simulink model "wamjc7"  (Simulink 8.3)
settings: Solver=ode4  SolverMode=SingleTasking  StartTime=0.0  StopTime=inf  FixedStep=sample_time  RelTol=1e-3
undefined symbols (not defined in the file): arm_home, arm_home_norest, arm_j2mt, arm_m2jp, b, bit, C, CAN_init, enc_per_rev, FT_init, hand_on, MT_init, puck_I_per_Nm, rotFT2Hand, sample_time, Standard, VL1_init, VL2_init
libraries: xpclib x43, simulink x27, xpcutilitieslib x6, dspmathops x1, dspadpt3 x1, dspindex x1, dspbuff3 x1
(part 5 of 5)

== matlab function Subsystem/Impedance Controller/Subsystem1/Dynamics Compensation1 ==
  data: hand_on input double; tau output double; q input double; qd input double; qdd input double; FTsensor output double
function [tau, FTsensor] = dynamicsComp(hand_on,q,qd,qdd)
%-------------------------------------------------------------------------------------
%   SETUP THE ARM
%-------------------------------------------------------------------------------------    
    DH_a = [0 0 0.045 -0.045 0 0 0];
    DH_d = [0 0 .55 0 0.3 0 0.061];
    DH_alpha = [-pi/2 pi/2 -pi/2 pi/2 -pi/2 pi/2 0];

    m = [8.3936 4.8487 1.7251 2.17266212 0.35655692 0.40915886 0.07548270];
    
    com = zeros(3,7);
    com(:,1) = [0.3506e-3, 132.6795e-3, 0.6286e-3];
    com(:,2) = [-0.2230e-3, -21.3924e-3, 13.3754e-3];
    com(:,3) = [-38.7565e-3, 217.9078e-3, 0.0252e-3];
    com(:,4) = [0.00553408,0.00006822,0.11927695];
    com(:,5) = [0.00005483,0.02886286,0.00148493];
    com(:,6) = [-0.00005923,-0.01686123,0.02419052];
    com(:,7) = [ 0.00014836,0.00007252,-0.00335185];
    
    % Need Inertia matricies
    I = zeros(3,3,7);
    I(:,:,1) = [ 95157.4294e-6,   246.1404e-6,   -95.0183e-6 ;
                   246.1404e-6, 92032.3524e-6,  -962.6725e-6 ;
                   -95.0183e-6,  -962.6725e-6, 59290.5997e-6 ];
    I(:,:,2) = [ 29326.8098e-6,   -43.3994e-6,  -129.2942e-6 ;
                   -43.3994e-6, 20781.5826e-6,  1348.6924e-6 ;
                  -129.2942e-6,  1348.6924e-6, 22807.3271e-6 ];
    I(:,:,3) = [ 56662.2970e-6, -2321.6892e-6,     8.2125e-6 ;
                 -2321.6892e-6,  3158.0509e-6,   -16.6307e-6 ;
                     8.2125e-6,   -16.6307e-6, 56806.6024e-6 ];
    I(:,:,4) = [  0.01067491,  0.00004503, -0.00135557 ;
                  0.00004503,  0.01058659, -0.00011002 ;
                 -0.00135557, -0.00011002,  0.00282036 ];
    I(:,:,5) = [  0.00037112, -0.00000008, -0.00000003 ;
                 -0.00000008,  0.00019434, -0.00001613 ;
                 -0.00000003, -0.00001613,  0.00038209 ];
    I(:,:,6) =  [  0.00054889,  0.00000019, -0.00000010 ;
                   0.00000019,  0.00023846, -0.00004430 ;
                  -0.00000010, -0.00004430,  0.00045133 ];
    I(:,:,7) = [ 0.00003911, 0.00000019, 0.00000000 ;      % WAM without hand
                 0.00000019, 0.00003877, 0.00000000 ;
                 0.00000000, 0.00000000, 0.00007614 ];
    
    %Link Gear Ratio
    % The differential drive mechanism was ignored here because it's not
    % supported by the robotic toolbox yet.
    % Please refer to: http://www.me.unm.edu/~starr/research/WAM_MassParams_AA-00.pdf
    G = zeros(7,1);
    G(1) =  42.00;
    G(2) =  28.25;
    G(3) =  28.25;
    G(4) =  18.00;
    G(5) =  9.70;
    G(6) =  9.70;
    G(7) =  14.93;
    %Link Motor Inertia
    Jm = zeros(7,1);
    Jm(1) = 0.00011631;
    Jm(2) = 0.00011831;
    Jm(3) = 0.00011831;
    Jm(4) = 0.00010686;
    Jm(5) = 0.00001685;
    Jm(6) = 0.00001745;
    Jm(7) = 0.00000142;
             
    if hand_on
        hand_mass = 1.3731;
        DH_d(7) = DH_d(7) + .0953; % Adding the distance to the hand frame for the Schunk Gripper
        com(:,7) = ([0.001127;	-0.000211;	0.054851].*hand_mass + com(:,7).*m(7))/(hand_mass + m(7)); % Finding the combined center of mass
        m(7) = m(7) + hand_mass; % Adding the mass of the hand
        I(:,:,7) = [ .003167342,          0,         0;       % Approximate Inertia Tensor for Schunk Gripper
                              0, .001128942,         0;
                              0,          0, .00258007;];
    end
    
%-------------------------------------------------------------------------------------
%  END SETUP OF THE ARM
%-------------------------------------------------------------------------------------

    z0 = [0;0;1];
    grav = [0 0 9.81];
	fext = zeros(6, 1);
    n = 7;
    FTsensor = zeros(6,1);
    
    tau = zeros(n,1);
    
    Fm = zeros(3,7);
    Nm = zeros(3,7);
    N = zeros(3,1);
    pstarm = zeros(3,7);
    Rm = zeros(3,3,7);
    w = zeros(3,1);
    wd = zeros(3,1);
    v = zeros(3,1);
    vd = grav(:);
    
    
    %
	% init some variables, compute the link rotation matrices
	%
    for j=1:n,
        a = DH_a(j);
        d = DH_d(j);
        alpha = DH_alpha(j);
        Tj = getTransformDH(a, d, alpha, q(j));
        
        pstar = [a; d*sin(alpha); d*cos(alpha)];
        if j == 1,
            pstar = eye(3) * pstar;
            Tj = eye(4) * Tj;
        end
        pstarm(:,j) = pstar;
        Rm(:,:,j) = Tj(1:3,1:3);
    end
    
    %
	%  the forward recursion
	%
    for j=1:n,
        Rt = Rm(:,:,j)';	% transpose!!
        pstar = pstarm(:,j);
        r = com(:,j)';

        %
        % statement order is important here
        %
        % revolute axis
        wd = Rt*(wd + z0*qdd(j) + cross(w,z0*qd(j)));
        w = Rt*(w + z0*qd(j));
        %v = cross(w,pstar) + Rt*v;
        vd = cross(wd,pstar) + cross(w, cross(w,pstar)) + Rt*vd;

        %vhat = cross(wd,r') + cross(w,cross(w,r')) + vd;
        vhat = cross(wd,r') + cross(w,cross(w,r')) + vd;
        F = m(j)*vhat;
        N = I(1:3,1:3,j)*wd + cross(w,I(1:3,1:3,j)*w);
        Fm(:,j) = F;
        Nm(:,j) = N;
    end
    
    
    %
	%  the backward recursion
	%

    fext = fext(:);
    f = fext(1:3);		% force/moments on end of arm
    nn = fext(4:6);

    for j=n:-1:1,
        pstar = pstarm(:,j);

        %
        % order of these statements is important, since both
        % nn and f are functions of previous f.
        %
        if j == n,
            R = eye(3,3);
        else
            R = Rm(:,:,j+1);
        end
        r = com(:,j)';
        
        % The expected force/torque at the sensor.  Used for dynamic compensation
        % of the gripper.
        if j == n
            FTsensor(1:3) = R*f + Fm(:,j);
            FTsensor(4:6) = cross(r',Fm(:,j));
        end
        
        nn = R*(nn + cross(R'*pstar,f)) + cross(pstar+r',Fm(:,j)) + Nm(:,j);
        f = R*f + Fm(:,j);
        
        R = Rm(:,:,j);
        % revolute
        tau(j) = nn'*(R'*z0) + G(j)^2 * Jm(j)*qdd(j);% + abs(G(j)) * friction(link, qd(j));
    end

end

function T = getTransformDH(a,d,alpha,q)
    ct = cos(q);
    st = sin(q);
    cb = cos(alpha);
    sb = sin(alpha);
    
    T = [ ct, -st*cb,  st*sb, a*ct;
          st,  ct*cb, -ct*sb, a*st;
          0, sb, cb, d;
          0, 0, 0, 1 ];
end

== matlab function Subsystem/Impedance Controller/Subsystem1/Dynamics Compensation2 ==
  data: hand_on input double; tau output double; q input double; qd input double; qdd input double; FTsensor output double
function [tau, FTsensor] = dynamicsComp(hand_on,q,qd,qdd)
%-------------------------------------------------------------------------------------
%   SETUP THE ARM
%-------------------------------------------------------------------------------------    
    DH_a = [0 0 0.045 -0.045 0 0 0];
    DH_d = [0 0 .55 0 0.3 0 0.061];
    DH_alpha = [-pi/2 pi/2 -pi/2 pi/2 -pi/2 pi/2 0];

    m = [8.3936 4.8487 1.7251 2.17266212 0.35655692 0.40915886 0.07548270];
    
    com = zeros(3,7);
    com(:,1) = [0.3506e-3, 132.6795e-3, 0.6286e-3];
    com(:,2) = [-0.2230e-3, -21.3924e-3, 13.3754e-3];
    com(:,3) = [-38.7565e-3, 217.9078e-3, 0.0252e-3];
    com(:,4) = [0.00553408,0.00006822,0.11927695];
    com(:,5) = [0.00005483,0.02886286,0.00148493];
    com(:,6) = [-0.00005923,-0.01686123,0.02419052];
    com(:,7) = [ 0.00014836,0.00007252,-0.00335185];
    
    % Need Inertia matricies
    I = zeros(3,3,7);
    I(:,:,1) = [ 95157.4294e-6,   246.1404e-6,   -95.0183e-6 ;
                   246.1404e-6, 92032.3524e-6,  -962.6725e-6 ;
                   -95.0183e-6,  -962.6725e-6, 59290.5997e-6 ];
    I(:,:,2) = [ 29326.8098e-6,   -43.3994e-6,  -129.2942e-6 ;
                   -43.3994e-6, 20781.5826e-6,  1348.6924e-6 ;
                  -129.2942e-6,  1348.6924e-6, 22807.3271e-6 ];
    I(:,:,3) = [ 56662.2970e-6, -2321.6892e-6,     8.2125e-6 ;
                 -2321.6892e-6,  3158.0509e-6,   -16.6307e-6 ;
                     8.2125e-6,   -16.6307e-6, 56806.6024e-6 ];
    I(:,:,4) = [  0.01067491,  0.00004503, -0.00135557 ;
                  0.00004503,  0.01058659, -0.00011002 ;
                 -0.00135557, -0.00011002,  0.00282036 ];
    I(:,:,5) = [  0.00037112, -0.00000008, -0.00000003 ;
                 -0.00000008,  0.00019434, -0.00001613 ;
                 -0.00000003, -0.00001613,  0.00038209 ];
    I(:,:,6) =  [  0.00054889,  0.00000019, -0.00000010 ;
                   0.00000019,  0.00023846, -0.00004430 ;
                  -0.00000010, -0.00004430,  0.00045133 ];
    I(:,:,7) = [ 0.00003911, 0.00000019, 0.00000000 ;      % WAM without hand
                 0.00000019, 0.00003877, 0.00000000 ;
                 0.00000000, 0.00000000, 0.00007614 ];
    
    %Link Gear Ratio
    % The differential drive mechanism was ignored here because it's not
    % supported by the robotic toolbox yet.
    % Please refer to: http://www.me.unm.edu/~starr/research/WAM_MassParams_AA-00.pdf
    G = zeros(7,1);
    G(1) =  42.00;
    G(2) =  28.25;
    G(3) =  28.25;
    G(4) =  18.00;
    G(5) =  9.70;
    G(6) =  9.70;
    G(7) =  14.93;
    %Link Motor Inertia
    Jm = zeros(7,1);
    Jm(1) = 0.00011631;
    Jm(2) = 0.00011831;
    Jm(3) = 0.00011831;
    Jm(4) = 0.00010686;
    Jm(5) = 0.00001685;
    Jm(6) = 0.00001745;
    Jm(7) = 0.00000142;
             
    if hand_on
        hand_mass = 1.3731;
        DH_d(7) = DH_d(7) + .0953; % Adding the distance to the hand frame for the Schunk Gripper
        com(:,7) = ([0.001127;	-0.000211;	0.054851].*hand_mass + com(:,7).*m(7))/(hand_mass + m(7)); % Finding the combined center of mass
        m(7) = m(7) + hand_mass; % Adding the mass of the hand
        I(:,:,7) = [ .003167342,          0,         0;       % Approximate Inertia Tensor for Schunk Gripper
                              0, .001128942,         0;
                              0,          0, .00258007;];
    end
    
%-------------------------------------------------------------------------------------
%  END SETUP OF THE ARM
%-------------------------------------------------------------------------------------

    z0 = [0;0;1];
    grav = [0 0 9.81];
	fext = zeros(6, 1);
    n = 7;
    FTsensor = zeros(6,1);
    
    tau = zeros(n,1);
    
    Fm = zeros(3,7);
    Nm = zeros(3,7);
    N = zeros(3,1);
    pstarm = zeros(3,7);
    Rm = zeros(3,3,7);
    w = zeros(3,1);
    wd = zeros(3,1);
    v = zeros(3,1);
    vd = grav(:);
    
    
    %
	% init some variables, compute the link rotation matrices
	%
    for j=1:n,
        a = DH_a(j);
        d = DH_d(j);
        alpha = DH_alpha(j);
        Tj = getTransformDH(a, d, alpha, q(j));
        
        pstar = [a; d*sin(alpha); d*cos(alpha)];
        if j == 1,
            pstar = eye(3) * pstar;
            Tj = eye(4) * Tj;
        end
        pstarm(:,j) = pstar;
        Rm(:,:,j) = Tj(1:3,1:3);
    end
    
    %
	%  the forward recursion
	%
    for j=1:n,
        Rt = Rm(:,:,j)';	% transpose!!
        pstar = pstarm(:,j);
        r = com(:,j)';

        %
        % statement order is important here
        %
        % revolute axis
        wd = Rt*(wd + z0*qdd(j) + cross(w,z0*qd(j)));
        w = Rt*(w + z0*qd(j));
        %v = cross(w,pstar) + Rt*v;
        vd = cross(wd,pstar) + cross(w, cross(w,pstar)) + Rt*vd;

        %vhat = cross(wd,r') + cross(w,cross(w,r')) + vd;
        vhat = cross(wd,r') + cross(w,cross(w,r')) + vd;
        F = m(j)*vhat;
        N = I(1:3,1:3,j)*wd + cross(w,I(1:3,1:3,j)*w);
        Fm(:,j) = F;
        Nm(:,j) = N;
    end
    
    
    %
	%  the backward recursion
	%

    fext = fext(:);
    f = fext(1:3);		% force/moments on end of arm
    nn = fext(4:6);

    for j=n:-1:1,
        pstar = pstarm(:,j);

        %
        % order of these statements is important, since both
        % nn and f are functions of previous f.
        %
        if j == n,
            R = eye(3,3);
        else
            R = Rm(:,:,j+1);
        end
        r = com(:,j)';
        
        % The expected force/torque at the sensor.  Used for dynamic compensation
        % of the gripper.
        if j == n
            FTsensor(1:3) = R*f + Fm(:,j);
            FTsensor(4:6) = cross(r',Fm(:,j));
        end
        
        nn = R*(nn + cross(R'*pstar,f)) + cross(pstar+r',Fm(:,j)) + Nm(:,j);
        f = R*f + Fm(:,j);
        
        R = Rm(:,:,j);
        % revolute
        tau(j) = nn'*(R'*z0) + G(j)^2 * Jm(j)*qdd(j);% + abs(G(j)) * friction(link, qd(j));
    end

end

function T = getTransformDH(a,d,alpha,q)
    ct = cos(q);
    st = sin(q);
    cb = cos(alpha);
    sb = sin(alpha);
    
    T = [ ct, -st*cb,  st*sb, a*ct;
          st,  ct*cb, -ct*sb, a*st;
          0, sb, cb, d;
          0, 0, 0, 1 ];
end

== matlab function Subsystem/Impedance Controller/Subsystem1/Dynamics Compensation3 ==
  data: hand_on input double; tau output double; q input double; qd input double; qdd input double; FTsensor output double
function [tau, FTsensor] = dynamicsComp(hand_on,q,qd,qdd)
%-------------------------------------------------------------------------------------
%   SETUP THE ARM
%-------------------------------------------------------------------------------------    
    DH_a = [0 0 0.045 -0.045 0 0 0];
    DH_d = [0 0 .55 0 0.3 0 0.061];
    DH_alpha = [-pi/2 pi/2 -pi/2 pi/2 -pi/2 pi/2 0];

    m = [8.3936 4.8487 1.7251 2.17266212 0.35655692 0.40915886 0.07548270];
    
    com = zeros(3,7);
    com(:,1) = [0.3506e-3, 132.6795e-3, 0.6286e-3];
    com(:,2) = [-0.2230e-3, -21.3924e-3, 13.3754e-3];
    com(:,3) = [-38.7565e-3, 217.9078e-3, 0.0252e-3];
    com(:,4) = [0.00553408,0.00006822,0.11927695];
    com(:,5) = [0.00005483,0.02886286,0.00148493];
    com(:,6) = [-0.00005923,-0.01686123,0.02419052];
    com(:,7) = [ 0.00014836,0.00007252,-0.00335185];
    
    % Need Inertia matricies
    I = zeros(3,3,7);
    I(:,:,1) = [ 95157.4294e-6,   246.1404e-6,   -95.0183e-6 ;
                   246.1404e-6, 92032.3524e-6,  -962.6725e-6 ;
                   -95.0183e-6,  -962.6725e-6, 59290.5997e-6 ];
    I(:,:,2) = [ 29326.8098e-6,   -43.3994e-6,  -129.2942e-6 ;
                   -43.3994e-6, 20781.5826e-6,  1348.6924e-6 ;
                  -129.2942e-6,  1348.6924e-6, 22807.3271e-6 ];
    I(:,:,3) = [ 56662.2970e-6, -2321.6892e-6,     8.2125e-6 ;
                 -2321.6892e-6,  3158.0509e-6,   -16.6307e-6 ;
                     8.2125e-6,   -16.6307e-6, 56806.6024e-6 ];
    I(:,:,4) = [  0.01067491,  0.00004503, -0.00135557 ;
                  0.00004503,  0.01058659, -0.00011002 ;
                 -0.00135557, -0.00011002,  0.00282036 ];
    I(:,:,5) = [  0.00037112, -0.00000008, -0.00000003 ;
                 -0.00000008,  0.00019434, -0.00001613 ;
                 -0.00000003, -0.00001613,  0.00038209 ];
    I(:,:,6) =  [  0.00054889,  0.00000019, -0.00000010 ;
                   0.00000019,  0.00023846, -0.00004430 ;
                  -0.00000010, -0.00004430,  0.00045133 ];
    I(:,:,7) = [ 0.00003911, 0.00000019, 0.00000000 ;      % WAM without hand
                 0.00000019, 0.00003877, 0.00000000 ;
                 0.00000000, 0.00000000, 0.00007614 ];
    
    %Link Gear Ratio
    % The differential drive mechanism was ignored here because it's not
    % supported by the robotic toolbox yet.
    % Please refer to: http://www.me.unm.edu/~starr/research/WAM_MassParams_AA-00.pdf
    G = zeros(7,1);
    G(1) =  42.00;
    G(2) =  28.25;
    G(3) =  28.25;
    G(4) =  18.00;
    G(5) =  9.70;
    G(6) =  9.70;
    G(7) =  14.93;
    %Link Motor Inertia
    Jm = zeros(7,1);
    Jm(1) = 0.00011631;
    Jm(2) = 0.00011831;
    Jm(3) = 0.00011831;
    Jm(4) = 0.00010686;
    Jm(5) = 0.00001685;
    Jm(6) = 0.00001745;
    Jm(7) = 0.00000142;
             
    if hand_on
        hand_mass = 1.3731;
        DH_d(7) = DH_d(7) + .0953; % Adding the distance to the hand frame for the Schunk Gripper
        com(:,7) = ([0.001127;	-0.000211;	0.054851].*hand_mass + com(:,7).*m(7))/(hand_mass + m(7)); % Finding the combined center of mass
        m(7) = m(7) + hand_mass; % Adding the mass of the hand
        I(:,:,7) = [ .003167342,          0,         0;       % Approximate Inertia Tensor for Schunk Gripper
                              0, .001128942,         0;
                              0,          0, .00258007;];
    end
    
%-------------------------------------------------------------------------------------
%  END SETUP OF THE ARM
%-------------------------------------------------------------------------------------

    z0 = [0;0;1];
    grav = [0 0 9.81];
	fext = zeros(6, 1);
    n = 7;
    FTsensor = zeros(6,1);
    
    tau = zeros(n,1);
    
    Fm = zeros(3,7);
    Nm = zeros(3,7);
    N = zeros(3,1);
    pstarm = zeros(3,7);
    Rm = zeros(3,3,7);
    w = zeros(3,1);
    wd = zeros(3,1);
    v = zeros(3,1);
    vd = grav(:);
    
    
    %
	% init some variables, compute the link rotation matrices
	%
    for j=1:n,
        a = DH_a(j);
        d = DH_d(j);
        alpha = DH_alpha(j);
        Tj = getTransformDH(a, d, alpha, q(j));
        
        pstar = [a; d*sin(alpha); d*cos(alpha)];
        if j == 1,
            pstar = eye(3) * pstar;
            Tj = eye(4) * Tj;
        end
        pstarm(:,j) = pstar;
        Rm(:,:,j) = Tj(1:3,1:3);
    end
    
    %
	%  the forward recursion
	%
    for j=1:n,
        Rt = Rm(:,:,j)';	% transpose!!
        pstar = pstarm(:,j);
        r = com(:,j)';

        %
        % statement order is important here
        %
        % revolute axis
        wd = Rt*(wd + z0*qdd(j) + cross(w,z0*qd(j)));
        w = Rt*(w + z0*qd(j));
        %v = cross(w,pstar) + Rt*v;
        vd = cross(wd,pstar) + cross(w, cross(w,pstar)) + Rt*vd;

        %vhat = cross(wd,r') + cross(w,cross(w,r')) + vd;
        vhat = cross(wd,r') + cross(w,cross(w,r')) + vd;
        F = m(j)*vhat;
        N = I(1:3,1:3,j)*wd + cross(w,I(1:3,1:3,j)*w);
        Fm(:,j) = F;
        Nm(:,j) = N;
    end
    
    
    %
	%  the backward recursion
	%

    fext = fext(:);
    f = fext(1:3);		% force/moments on end of arm
    nn = fext(4:6);

    for j=n:-1:1,
        pstar = pstarm(:,j);

        %
        % order of these statements is important, since both
        % nn and f are functions of previous f.
        %
        if j == n,
            R = eye(3,3);
        else
            R = Rm(:,:,j+1);
        end
        r = com(:,j)';
        
        % The expected force/torque at the sensor.  Used for dynamic compensation
        % of the gripper.
        if j == n
            FTsensor(1:3) = R*f + Fm(:,j);
            FTsensor(4:6) = cross(r',Fm(:,j));
        end
        
        nn = R*(nn + cross(R'*pstar,f)) + cross(pstar+r',Fm(:,j)) + Nm(:,j);
        f = R*f + Fm(:,j);
        
        R = Rm(:,:,j);
        % revolute
        tau(j) = nn'*(R'*z0) + G(j)^2 * Jm(j)*qdd(j);% + abs(G(j)) * friction(link, qd(j));
    end

end

function T = getTransformDH(a,d,alpha,q)
    ct = cos(q);
    st = sin(q);
    cb = cos(alpha);
    sb = sin(alpha);
    
    T = [ ct, -st*cb,  st*sb, a*ct;
          st,  ct*cb, -ct*sb, a*st;
          0, sb, cb, d;
          0, 0, 0, 1 ];
end

== matlab function Subsystem/Impedance Controller/Subsystem1/Dynamics Compensation4 ==
  data: hand_on input double; tau output double; q input double; qd input double; qdd input double; FTsensor output double
function [tau, FTsensor] = dynamicsComp(hand_on,q,qd,qdd)
%-------------------------------------------------------------------------------------
%   SETUP THE ARM
%-------------------------------------------------------------------------------------    
    DH_a = [0 0 0.045 -0.045 0 0 0];
    DH_d = [0 0 .55 0 0.3 0 0.061];
    DH_alpha = [-pi/2 pi/2 -pi/2 pi/2 -pi/2 pi/2 0];

    m = [8.3936 4.8487 1.7251 2.17266212 0.35655692 0.40915886 0.07548270];
    
    com = zeros(3,7);
    com(:,1) = [0.3506e-3, 132.6795e-3, 0.6286e-3];
    com(:,2) = [-0.2230e-3, -21.3924e-3, 13.3754e-3];
    com(:,3) = [-38.7565e-3, 217.9078e-3, 0.0252e-3];
    com(:,4) = [0.00553408,0.00006822,0.11927695];
    com(:,5) = [0.00005483,0.02886286,0.00148493];
    com(:,6) = [-0.00005923,-0.01686123,0.02419052];
    com(:,7) = [ 0.00014836,0.00007252,-0.00335185];
    
    % Need Inertia matricies
    I = zeros(3,3,7);
    I(:,:,1) = [ 95157.4294e-6,   246.1404e-6,   -95.0183e-6 ;
                   246.1404e-6, 92032.3524e-6,  -962.6725e-6 ;
                   -95.0183e-6,  -962.6725e-6, 59290.5997e-6 ];
    I(:,:,2) = [ 29326.8098e-6,   -43.3994e-6,  -129.2942e-6 ;
                   -43.3994e-6, 20781.5826e-6,  1348.6924e-6 ;
                  -129.2942e-6,  1348.6924e-6, 22807.3271e-6 ];
    I(:,:,3) = [ 56662.2970e-6, -2321.6892e-6,     8.2125e-6 ;
                 -2321.6892e-6,  3158.0509e-6,   -16.6307e-6 ;
                     8.2125e-6,   -16.6307e-6, 56806.6024e-6 ];
    I(:,:,4) = [  0.01067491,  0.00004503, -0.00135557 ;
                  0.00004503,  0.01058659, -0.00011002 ;
                 -0.00135557, -0.00011002,  0.00282036 ];
    I(:,:,5) = [  0.00037112, -0.00000008, -0.00000003 ;
                 -0.00000008,  0.00019434, -0.00001613 ;
                 -0.00000003, -0.00001613,  0.00038209 ];
    I(:,:,6) =  [  0.00054889,  0.00000019, -0.00000010 ;
                   0.00000019,  0.00023846, -0.00004430 ;
                  -0.00000010, -0.00004430,  0.00045133 ];
    I(:,:,7) = [ 0.00003911, 0.00000019, 0.00000000 ;      % WAM without hand
                 0.00000019, 0.00003877, 0.00000000 ;
                 0.00000000, 0.00000000, 0.00007614 ];
    
    %Link Gear Ratio
    % The differential drive mechanism was ignored here because it's not
    % supported by the robotic toolbox yet.
    % Please refer to: http://www.me.unm.edu/~starr/research/WAM_MassParams_AA-00.pdf
    G = zeros(7,1);
    G(1) =  42.00;
    G(2) =  28.25;
    G(3) =  28.25;
    G(4) =  18.00;
    G(5) =  9.70;
    G(6) =  9.70;
    G(7) =  14.93;
    %Link Motor Inertia
    Jm = zeros(7,1);
    Jm(1) = 0.00011631;
    Jm(2) = 0.00011831;
    Jm(3) = 0.00011831;
    Jm(4) = 0.00010686;
    Jm(5) = 0.00001685;
    Jm(6) = 0.00001745;
    Jm(7) = 0.00000142;
             
    if hand_on
        hand_mass = 1.3731;
        DH_d(7) = DH_d(7) + .0953; % Adding the distance to the hand frame for the Schunk Gripper
        com(:,7) = ([0.001127;	-0.000211;	0.054851].*hand_mass + com(:,7).*m(7))/(hand_mass + m(7)); % Finding the combined center of mass
        m(7) = m(7) + hand_mass; % Adding the mass of the hand
        I(:,:,7) = [ .003167342,          0,         0;       % Approximate Inertia Tensor for Schunk Gripper
                              0, .001128942,         0;
                              0,          0, .00258007;];
    end
    
%-------------------------------------------------------------------------------------
%  END SETUP OF THE ARM
%-------------------------------------------------------------------------------------

    z0 = [0;0;1];
    grav = [0 0 9.81];
	fext = zeros(6, 1);
    n = 7;
    FTsensor = zeros(6,1);
    
    tau = zeros(n,1);
    
    Fm = zeros(3,7);
    Nm = zeros(3,7);
    N = zeros(3,1);
    pstarm = zeros(3,7);
    Rm = zeros(3,3,7);
    w = zeros(3,1);
    wd = zeros(3,1);
    v = zeros(3,1);
    vd = grav(:);
    
    
    %
	% init some variables, compute the link rotation matrices
	%
    for j=1:n,
        a = DH_a(j);
        d = DH_d(j);
        alpha = DH_alpha(j);
        Tj = getTransformDH(a, d, alpha, q(j));
        
        pstar = [a; d*sin(alpha); d*cos(alpha)];
        if j == 1,
            pstar = eye(3) * pstar;
            Tj = eye(4) * Tj;
        end
        pstarm(:,j) = pstar;
        Rm(:,:,j) = Tj(1:3,1:3);
    end
    
    %
	%  the forward recursion
	%
    for j=1:n,
        Rt = Rm(:,:,j)';	% transpose!!
        pstar = pstarm(:,j);
        r = com(:,j)';

        %
        % statement order is important here
        %
        % revolute axis
        wd = Rt*(wd + z0*qdd(j) + cross(w,z0*qd(j)));
        w = Rt*(w + z0*qd(j));
        %v = cross(w,pstar) + Rt*v;
        vd = cross(wd,pstar) + cross(w, cross(w,pstar)) + Rt*vd;

        %vhat = cross(wd,r') + cross(w,cross(w,r')) + vd;
        vhat = cross(wd,r') + cross(w,cross(w,r')) + vd;
        F = m(j)*vhat;
        N = I(1:3,1:3,j)*wd + cross(w,I(1:3,1:3,j)*w);
        Fm(:,j) = F;
        Nm(:,j) = N;
    end
    
    
    %
	%  the backward recursion
	%

    fext = fext(:);
    f = fext(1:3);		% force/moments on end of arm
    nn = fext(4:6);

    for j=n:-1:1,
        pstar = pstarm(:,j);

        %
        % order of these statements is important, since both
        % nn and f are functions of previous f.
        %
        if j == n,
            R = eye(3,3);
        else
            R = Rm(:,:,j+1);
        end
        r = com(:,j)';
        
        % The expected force/torque at the sensor.  Used for dynamic compensation
        % of the gripper.
        if j == n
            FTsensor(1:3) = R*f + Fm(:,j);
            FTsensor(4:6) = cross(r',Fm(:,j));
        end
        
        nn = R*(nn + cross(R'*pstar,f)) + cross(pstar+r',Fm(:,j)) + Nm(:,j);
        f = R*f + Fm(:,j);
        
        R = Rm(:,:,j);
        % revolute
        tau(j) = nn'*(R'*z0) + G(j)^2 * Jm(j)*qdd(j);% + abs(G(j)) * friction(link, qd(j));
    end

end

function T = getTransformDH(a,d,alpha,q)
    ct = cos(q);
    st = sin(q);
    cb = cos(alpha);
    sb = sin(alpha);
    
    T = [ ct, -st*cb,  st*sb, a*ct;
          st,  ct*cb, -ct*sb, a*st;
          0, sb, cb, d;
          0, 0, 0, 1 ];
end

== matlab function Subsystem/Impedance Controller/Subsystem1/Dynamics Compensation5 ==
  data: hand_on input double; tau output double; q input double; qd input double; qdd input double; FTsensor output double
function [tau, FTsensor] = dynamicsComp(hand_on,q,qd,qdd)
%-------------------------------------------------------------------------------------
%   SETUP THE ARM
%-------------------------------------------------------------------------------------    
    DH_a = [0 0 0.045 -0.045 0 0 0];
    DH_d = [0 0 .55 0 0.3 0 0.061];
    DH_alpha = [-pi/2 pi/2 -pi/2 pi/2 -pi/2 pi/2 0];

    m = [8.3936 4.8487 1.7251 2.17266212 0.35655692 0.40915886 0.07548270];
    
    com = zeros(3,7);
    com(:,1) = [0.3506e-3, 132.6795e-3, 0.6286e-3];
    com(:,2) = [-0.2230e-3, -21.3924e-3, 13.3754e-3];
    com(:,3) = [-38.7565e-3, 217.9078e-3, 0.0252e-3];
    com(:,4) = [0.00553408,0.00006822,0.11927695];
    com(:,5) = [0.00005483,0.02886286,0.00148493];
    com(:,6) = [-0.00005923,-0.01686123,0.02419052];
    com(:,7) = [ 0.00014836,0.00007252,-0.00335185];
    
    % Need Inertia matricies
    I = zeros(3,3,7);
    I(:,:,1) = [ 95157.4294e-6,   246.1404e-6,   -95.0183e-6 ;
                   246.1404e-6, 92032.3524e-6,  -962.6725e-6 ;
                   -95.0183e-6,  -962.6725e-6, 59290.5997e-6 ];
    I(:,:,2) = [ 29326.8098e-6,   -43.3994e-6,  -129.2942e-6 ;
                   -43.3994e-6, 20781.5826e-6,  1348.6924e-6 ;
                  -129.2942e-6,  1348.6924e-6, 22807.3271e-6 ];
    I(:,:,3) = [ 56662.2970e-6, -2321.6892e-6,     8.2125e-6 ;
                 -2321.6892e-6,  3158.0509e-6,   -16.6307e-6 ;
                     8.2125e-6,   -16.6307e-6, 56806.6024e-6 ];
    I(:,:,4) = [  0.01067491,  0.00004503, -0.00135557 ;
                  0.00004503,  0.01058659, -0.00011002 ;
                 -0.00135557, -0.00011002,  0.00282036 ];
    I(:,:,5) = [  0.00037112, -0.00000008, -0.00000003 ;
                 -0.00000008,  0.00019434, -0.00001613 ;
                 -0.00000003, -0.00001613,  0.00038209 ];
    I(:,:,6) =  [  0.00054889,  0.00000019, -0.00000010 ;
                   0.00000019,  0.00023846, -0.00004430 ;
                  -0.00000010, -0.00004430,  0.00045133 ];
    I(:,:,7) = [ 0.00003911, 0.00000019, 0.00000000 ;      % WAM without hand
                 0.00000019, 0.00003877, 0.00000000 ;
                 0.00000000, 0.00000000, 0.00007614 ];
    
    %Link Gear Ratio
    % The differential drive mechanism was ignored here because it's not
    % supported by the robotic toolbox yet.
    % Please refer to: http://www.me.unm.edu/~starr/research/WAM_MassParams_AA-00.pdf
    G = zeros(7,1);
    G(1) =  42.00;
    G(2) =  28.25;
    G(3) =  28.25;
    G(4) =  18.00;
    G(5) =  9.70;
    G(6) =  9.70;
    G(7) =  14.93;
    %Link Motor Inertia
    Jm = zeros(7,1);
    Jm(1) = 0.00011631;
    Jm(2) = 0.00011831;
    Jm(3) = 0.00011831;
    Jm(4) = 0.00010686;
    Jm(5) = 0.00001685;
    Jm(6) = 0.00001745;
    Jm(7) = 0.00000142;
             
    if hand_on
        hand_mass = 1.3731;
        DH_d(7) = DH_d(7) + .0953; % Adding the distance to the hand frame for the Schunk Gripper
        com(:,7) = ([0.001127;	-0.000211;	0.054851].*hand_mass + com(:,7).*m(7))/(hand_mass + m(7)); % Finding the combined center of mass
        m(7) = m(7) + hand_mass; % Adding the mass of the hand
        I(:,:,7) = [ .003167342,          0,         0;       % Approximate Inertia Tensor for Schunk Gripper
                              0, .001128942,         0;
                              0,          0, .00258007;];
    end
    
%-------------------------------------------------------------------------------------
%  END SETUP OF THE ARM
%-------------------------------------------------------------------------------------

    z0 = [0;0;1];
    grav = [0 0 9.81];
	fext = zeros(6, 1);
    n = 7;
    FTsensor = zeros(6,1);
    
    tau = zeros(n,1);
    
    Fm = zeros(3,7);
    Nm = zeros(3,7);
    N = zeros(3,1);
    pstarm = zeros(3,7);
    Rm = zeros(3,3,7);
    w = zeros(3,1);
    wd = zeros(3,1);
    v = zeros(3,1);
    vd = grav(:);
    
    
    %
	% init some variables, compute the link rotation matrices
	%
    for j=1:n,
        a = DH_a(j);
        d = DH_d(j);
        alpha = DH_alpha(j);
        Tj = getTransformDH(a, d, alpha, q(j));
        
        pstar = [a; d*sin(alpha); d*cos(alpha)];
        if j == 1,
            pstar = eye(3) * pstar;
            Tj = eye(4) * Tj;
        end
        pstarm(:,j) = pstar;
        Rm(:,:,j) = Tj(1:3,1:3);
    end
    
    %
	%  the forward recursion
	%
    for j=1:n,
        Rt = Rm(:,:,j)';	% transpose!!
        pstar = pstarm(:,j);
        r = com(:,j)';

        %
        % statement order is important here
        %
        % revolute axis
        wd = Rt*(wd + z0*qdd(j) + cross(w,z0*qd(j)));
        w = Rt*(w + z0*qd(j));
        %v = cross(w,pstar) + Rt*v;
        vd = cross(wd,pstar) + cross(w, cross(w,pstar)) + Rt*vd;

        %vhat = cross(wd,r') + cross(w,cross(w,r')) + vd;
        vhat = cross(wd,r') + cross(w,cross(w,r')) + vd;
        F = m(j)*vhat;
        N = I(1:3,1:3,j)*wd + cross(w,I(1:3,1:3,j)*w);
        Fm(:,j) = F;
        Nm(:,j) = N;
    end
    
    
    %
	%  the backward recursion
	%

    fext = fext(:);
    f = fext(1:3);		% force/moments on end of arm
    nn = fext(4:6);

    for j=n:-1:1,
        pstar = pstarm(:,j);

        %
        % order of these statements is important, since both
        % nn and f are functions of previous f.
        %
        if j == n,
            R = eye(3,3);
        else
            R = Rm(:,:,j+1);
        end
        r = com(:,j)';
        
        % The expected force/torque at the sensor.  Used for dynamic compensation
        % of the gripper.
        if j == n
            FTsensor(1:3) = R*f + Fm(:,j);
            FTsensor(4:6) = cross(r',Fm(:,j));
        end
        
        nn = R*(nn + cross(R'*pstar,f)) + cross(pstar+r',Fm(:,j)) + Nm(:,j);
        f = R*f + Fm(:,j);
        
        R = Rm(:,:,j);
        % revolute
        tau(j) = nn'*(R'*z0) + G(j)^2 * Jm(j)*qdd(j);% + abs(G(j)) * friction(link, qd(j));
    end

end

function T = getTransformDH(a,d,alpha,q)
    ct = cos(q);
    st = sin(q);
    cb = cos(alpha);
    sb = sin(alpha);
    
    T = [ ct, -st*cb,  st*sb, a*ct;
          st,  ct*cb, -ct*sb, a*st;
          0, sb, cb, d;
          0, 0, 0, 1 ];
end

== matlab function Subsystem/Impedance Controller/Subsystem1/Dynamics Compensation6 ==
  data: hand_on input double; tau output double; q input double; qd input double; qdd input double; FTsensor output double
function [tau, FTsensor] = dynamicsComp(hand_on,q,qd,qdd)
%-------------------------------------------------------------------------------------
%   SETUP THE ARM
%-------------------------------------------------------------------------------------    
    DH_a = [0 0 0.045 -0.045 0 0 0];
    DH_d = [0 0 .55 0 0.3 0 0.061];
    DH_alpha = [-pi/2 pi/2 -pi/2 pi/2 -pi/2 pi/2 0];

    m = [8.3936 4.8487 1.7251 2.17266212 0.35655692 0.40915886 0.07548270];
    
    com = zeros(3,7);
    com(:,1) = [0.3506e-3, 132.6795e-3, 0.6286e-3];
    com(:,2) = [-0.2230e-3, -21.3924e-3, 13.3754e-3];
    com(:,3) = [-38.7565e-3, 217.9078e-3, 0.0252e-3];
    com(:,4) = [0.00553408,0.00006822,0.11927695];
    com(:,5) = [0.00005483,0.02886286,0.00148493];
    com(:,6) = [-0.00005923,-0.01686123,0.02419052];
    com(:,7) = [ 0.00014836,0.00007252,-0.00335185];
    
    % Need Inertia matricies
    I = zeros(3,3,7);
    I(:,:,1) = [ 95157.4294e-6,   246.1404e-6,   -95.0183e-6 ;
                   246.1404e-6, 92032.3524e-6,  -962.6725e-6 ;
                   -95.0183e-6,  -962.6725e-6, 59290.5997e-6 ];
    I(:,:,2) = [ 29326.8098e-6,   -43.3994e-6,  -129.2942e-6 ;
                   -43.3994e-6, 20781.5826e-6,  1348.6924e-6 ;
                  -129.2942e-6,  1348.6924e-6, 22807.3271e-6 ];
    I(:,:,3) = [ 56662.2970e-6, -2321.6892e-6,     8.2125e-6 ;
                 -2321.6892e-6,  3158.0509e-6,   -16.6307e-6 ;
                     8.2125e-6,   -16.6307e-6, 56806.6024e-6 ];
    I(:,:,4) = [  0.01067491,  0.00004503, -0.00135557 ;
                  0.00004503,  0.01058659, -0.00011002 ;
                 -0.00135557, -0.00011002,  0.00282036 ];
    I(:,:,5) = [  0.00037112, -0.00000008, -0.00000003 ;
                 -0.00000008,  0.00019434, -0.00001613 ;
                 -0.00000003, -0.00001613,  0.00038209 ];
    I(:,:,6) =  [  0.00054889,  0.00000019, -0.00000010 ;
                   0.00000019,  0.00023846, -0.00004430 ;
                  -0.00000010, -0.00004430,  0.00045133 ];
    I(:,:,7) = [ 0.00003911, 0.00000019, 0.00000000 ;      % WAM without hand
                 0.00000019, 0.00003877, 0.00000000 ;
                 0.00000000, 0.00000000, 0.00007614 ];
    
    %Link Gear Ratio
    % The differential drive mechanism was ignored here because it's not
    % supported by the robotic toolbox yet.
    % Please refer to: http://www.me.unm.edu/~starr/research/WAM_MassParams_AA-00.pdf
    G = zeros(7,1);
    G(1) =  42.00;
    G(2) =  28.25;
    G(3) =  28.25;
    G(4) =  18.00;
    G(5) =  9.70;
    G(6) =  9.70;
    G(7) =  14.93;
    %Link Motor Inertia
    Jm = zeros(7,1);
    Jm(1) = 0.00011631;
    Jm(2) = 0.00011831;
    Jm(3) = 0.00011831;
    Jm(4) = 0.00010686;
    Jm(5) = 0.00001685;
    Jm(6) = 0.00001745;
    Jm(7) = 0.00000142;
             
    if hand_on
        hand_mass = 1.3731;
        DH_d(7) = DH_d(7) + .0953; % Adding the distance to the hand frame for the Schunk Gripper
        com(:,7) = ([0.001127;	-0.000211;	0.054851].*hand_mass + com(:,7).*m(7))/(hand_mass + m(7)); % Finding the combined center of mass
        m(7) = m(7) + hand_mass; % Adding the mass of the hand
        I(:,:,7) = [ .003167342,          0,         0;       % Approximate Inertia Tensor for Schunk Gripper
                              0, .001128942,         0;
                              0,          0, .00258007;];
    end
    
%-------------------------------------------------------------------------------------
%  END SETUP OF THE ARM
%-------------------------------------------------------------------------------------

    z0 = [0;0;1];
    grav = [0 0 9.81];
	fext = zeros(6, 1);
    n = 7;
    FTsensor = zeros(6,1);
    
    tau = zeros(n,1);
    
    Fm = zeros(3,7);
    Nm = zeros(3,7);
    N = zeros(3,1);
    pstarm = zeros(3,7);
    Rm = zeros(3,3,7);
    w = zeros(3,1);
    wd = zeros(3,1);
    v = zeros(3,1);
    vd = grav(:);
    
    
    %
	% init some variables, compute the link rotation matrices
	%
    for j=1:n,
        a = DH_a(j);
        d = DH_d(j);
        alpha = DH_alpha(j);
        Tj = getTransformDH(a, d, alpha, q(j));
        
        pstar = [a; d*sin(alpha); d*cos(alpha)];
        if j == 1,
            pstar = eye(3) * pstar;
            Tj = eye(4) * Tj;
        end
        pstarm(:,j) = pstar;
        Rm(:,:,j) = Tj(1:3,1:3);
    end
    
    %
	%  the forward recursion
	%
    for j=1:n,
        Rt = Rm(:,:,j)';	% transpose!!
        pstar = pstarm(:,j);
        r = com(:,j)';

        %
        % statement order is important here
        %
        % revolute axis
        wd = Rt*(wd + z0*qdd(j) + cross(w,z0*qd(j)));
        w = Rt*(w + z0*qd(j));
        %v = cross(w,pstar) + Rt*v;
        vd = cross(wd,pstar) + cross(w, cross(w,pstar)) + Rt*vd;

        %vhat = cross(wd,r') + cross(w,cross(w,r')) + vd;
        vhat = cross(wd,r') + cross(w,cross(w,r')) + vd;
        F = m(j)*vhat;
        N = I(1:3,1:3,j)*wd + cross(w,I(1:3,1:3,j)*w);
        Fm(:,j) = F;
        Nm(:,j) = N;
    end
    
    
    %
	%  the backward recursion
	%

    fext = fext(:);
    f = fext(1:3);		% force/moments on end of arm
    nn = fext(4:6);

    for j=n:-1:1,
        pstar = pstarm(:,j);

        %
        % order of these statements is important, since both
        % nn and f are functions of previous f.
        %
        if j == n,
            R = eye(3,3);
        else
            R = Rm(:,:,j+1);
        end
        r = com(:,j)';
        
        % The expected force/torque at the sensor.  Used for dynamic compensation
        % of the gripper.
        if j == n
            FTsensor(1:3) = R*f + Fm(:,j);
            FTsensor(4:6) = cross(r',Fm(:,j));
        end
        
        nn = R*(nn + cross(R'*pstar,f)) + cross(pstar+r',Fm(:,j)) + Nm(:,j);
        f = R*f + Fm(:,j);
        
        R = Rm(:,:,j);
        % revolute
        tau(j) = nn'*(R'*z0) + G(j)^2 * Jm(j)*qdd(j);% + abs(G(j)) * friction(link, qd(j));
    end

end

function T = getTransformDH(a,d,alpha,q)
    ct = cos(q);
    st = sin(q);
    cb = cos(alpha);
    sb = sin(alpha);
    
    T = [ ct, -st*cb,  st*sb, a*ct;
          st,  ct*cb, -ct*sb, a*st;
          0, sb, cb, d;
          0, 0, 0, 1 ];
end

== matlab function Get Arm State/Get Gripper Status/Grasp Success1 ==
  data: isMoveFingerMessage input double; axis_blocked output double; errorcode input double
function axis_blocked = f(isMoveFingerMessage, errorcode)
%#eml

    E_AXIS_BLOCKED = 29;

    persistent errorcode_last;
    
    if isempty(errorcode_last)
       errorcode_last = -1; 
    end

    axis_blocked = 0;
    
    % If this is a move finger message, whose error code is E_AXIS_BLOCKED and the last 
    % error code was not E_AXIS_BLOCKED retun a 1
    if isMoveFingerMessage && errorcode == E_AXIS_BLOCKED && errorcode_last ~= E_AXIS_BLOCKED
       axis_blocked = 1; 
       errorcode_last = double(errorcode);
    elseif ~isMoveFingerMessage
        errorcode_last = -1;
    end
end

== matlab function Subsystem/Plan Arm Trajectory/Embedded MATLAB Function ==
  data: FTError input double; Eout output double; contact_or_not input double; contact_scenario input double; Cout output double
function [Eout, Cout] = f(FTError, contact_or_not, contact_scenario)
%#eml

    persistent Esteps_remaining Csteps_remaining contact_or_not_first contact_scenario_first;
    
    Eout = zeros(3,1);
    Cout = zeros(2,1);

    if isempty(Esteps_remaining)
        Esteps_remaining = 0;
    end
    if isempty(Csteps_remaining)
        Csteps_remaining = 0;
    end
    if isempty(contact_or_not_first) || isempty(contact_scenario_first)
       contact_or_not_first = 0;
       contact_scenario_first = 0;
    end
    
    if FTError
       Esteps_remaining = 2;
    end
    if Esteps_remaining > 0
        Eout(1) = 1;
        Eout(2) = contact_or_not;
        Eout(3) = contact_scenario;
        Esteps_remaining = Esteps_remaining - 1;
    else
        Eout(1) = 0;
        Eout(2) = 0;
        Eout(3) = 0;
    end
    
    if contact_or_not > 0
        Csteps_remaining = 20;
        contact_or_not_first = contact_or_not;
        contact_scenario_first = contact_scenario;
    end
    if Csteps_remaining > 0
        Cout(1) = contact_or_not_first;
        Cout(2) = contact_scenario_first;
        Csteps_remaining = Csteps_remaining - 1;
    else
        contact_or_not_first = 0;
        contact_scenario_first = 0;
        Cout(1) = 0;
        Cout(2) = 0;
    end
    
end

== matlab function Subsystem/Impedance Controller/Convert NaN to Zero1 ==
  data: u input double; y output double
function y = fcn(u)
%#eml

u(isnan(u)) = 0; % convert NaN into 0!!!!

%uMax = [15.0 25.0 8.0 8.0 2.0 3.0 2.0];
uMax = [77.3 160.6 95.6 29.4 11.6 11.6 2.7]*.99;

for i = 1:7
   if u(i) < -uMax(i)
       u(i) = -uMax(i);
   end
   if u(i) > uMax(i)
       u(i) = uMax(i);
   end
end
   

y = u;

== matlab function Subsystem/Limit taud ==
  data: u input double; y output double
function y = fcn(u)
check = u>[2000 2000 2000 2000 2000 2000 2000]';

error = sum(check)>0;

if error
    y = 1;
else
    y = 0;
end

== matlab function Subsystem/Plan Arm Trajectory/Embedded MATLAB Function1 ==
  data: InContact input double; FTerr input double; ImpErr input double; ImpErrOut output double
function ImpErrOut  = f(InContact, FTerr,ImpErr)
%#eml
    
    ImpErr = double(ImpErr) || double(FTerr) || double(InContact);

    if ImpErr
        ImpErrOut = 1;
    else
        ImpErrOut = 0;
    end

end
